simulink subsystem "FCS"  (R2020a)
settings: Solver=VariableStepAuto  StartTime=0.0  StopTime=10.0  RelTol=1e-3
settings Model: Creator=Fatih  LastModifiedBy=Fatih

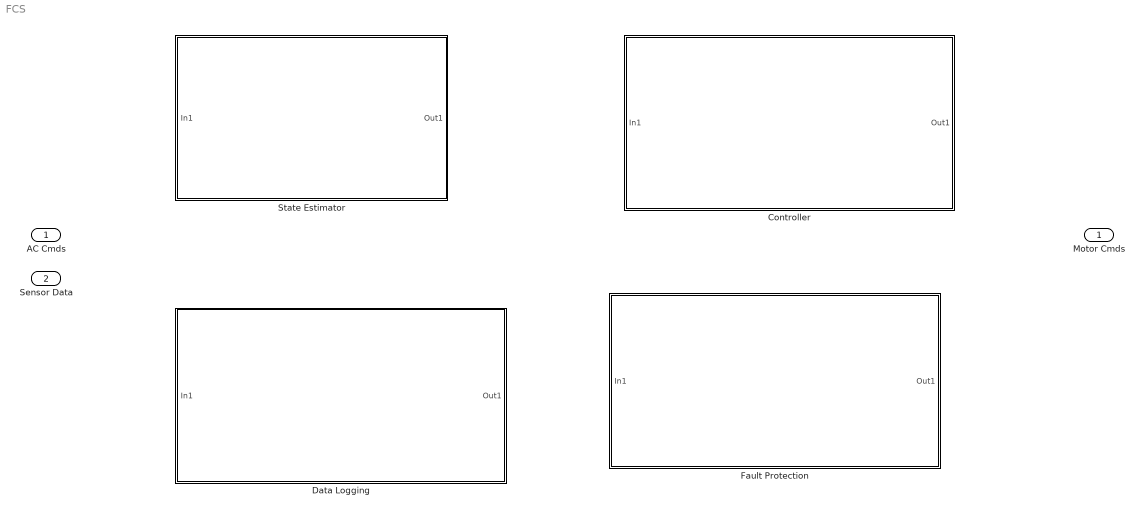
== system FCS ==
  AC Cmds : Inport
  Sensor Data : Inport  Port=2
  Controller : Subsystem
  Data Logging : Subsystem
  Fault Protection : Subsystem
  State Estimator : Subsystem
  Motor Cmds : Outport

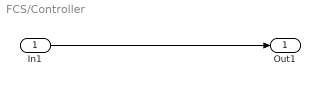
== system FCS/Controller ==
  In1 : Inport
  Out1 : Outport
  wires:
  In1/1 -> Out1/1

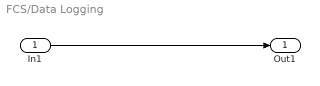
== system FCS/Data Logging ==
  In1 : Inport
  Out1 : Outport
  wires:
  In1/1 -> Out1/1

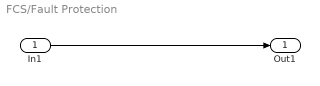
== system FCS/Fault Protection ==
  In1 : Inport
  Out1 : Outport
  wires:
  In1/1 -> Out1/1

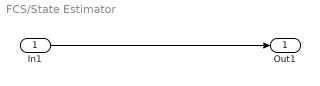
== system FCS/State Estimator ==
  In1 : Inport
  Out1 : Outport
  wires:
  In1/1 -> Out1/1
